simulink model "mini_car_ble"  (R2024a)
settings: Solver=FixedStepAuto  StartTime=0.0  StopTime=inf  FixedStep=0.02  RelTol=1e-3
undefined symbols (not defined in the file): u2, u3, u4, u5
libraries: simulink x57
settings Model: Creator=ext_matsmi1  LastModifiedBy=Matheus Smidi
settings OptimizationCC: DefaultParameterBehavior=Inlined  EnhancedBackFolding=on  PassReuseOutputArgsAs=Individual arguments  ZeroExternalMemoryAtStartup=off  ZeroInternalMemoryAtStartup=off  OptimizeBlockOrder=speed  DifferentSizesBufferReuse=on  OptimizationCustomize=off  EfficientTunableParamExpr=on
settings DebuggingCC: ParameterTunabilityLossMsg=error
settings HardwareCC: ProdHWDeviceType=AMD->x86-64 (Windows64)
settings SFSimCC: MATLABDynamicMemAlloc=off
settings RTWCC: Description=Embedded Coder  SystemTargetFile=ert.tlc  TemplateMakefile=ert_default_tmf  GPUComputeCapability=3.5
settings CodeAppCC: ForceParamTrailComments=on  IgnoreCustomStorageClasses=off  OperatorAnnotations=on  SimulinkDataObjDesc=on  SFDataObjDesc=on  InsertBlockDesc=on
settings ERTTargetCC: TargetLangStandard=C99 (ISO)  GenerateSampleERTMain=on  InlinedParameterPlacement=NonHierarchical  ERTCustomFileTemplate=example_file_process.tlc

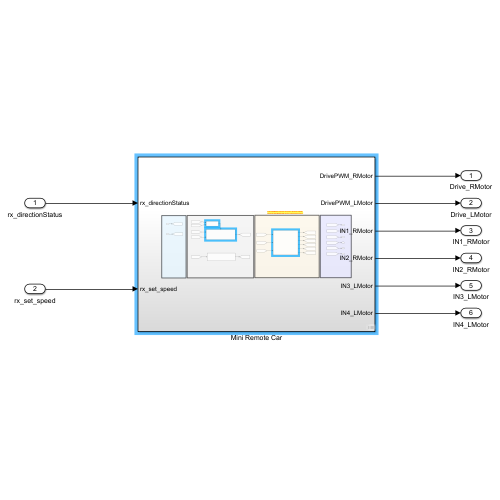
[thumbnail: Simulink's stored preview of the top-level diagram]
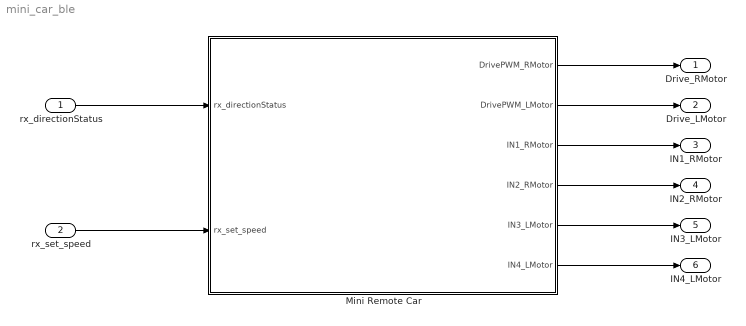
== system mini_car_ble ==
  rx_directionStatus : Inport  OutDataTypeStr=uint16
  rx_set_speed : Inport  Port=2  OutDataTypeStr=uint16
  Mini Remote Car : Subsystem
  Drive_RMotor : Outport
  Drive_LMotor : Outport  Port=2
  IN1_RMotor : Outport  Port=3
  IN2_RMotor : Outport  Port=4
  IN3_LMotor : Outport  Port=5
  IN4_LMotor : Outport  Port=6
  wires:
  Mini Remote Car/3(IN1_RMotor) -> IN1_RMotor/1
  Mini Remote Car/1(DrivePWM_RMotor) -> Drive_RMotor/1
  Mini Remote Car/6(IN4_LMotor) -> IN4_LMotor/1
  Mini Remote Car/4(IN2_RMotor) -> IN2_RMotor/1
  Mini Remote Car/5(IN3_LMotor) -> IN3_LMotor/1
  Mini Remote Car/2(DrivePWM_LMotor) -> Drive_LMotor/1
  rx_set_speed/1 -> Mini Remote Car/2(rx_set_speed)
  rx_directionStatus/1 -> Mini Remote Car/1(rx_directionStatus)

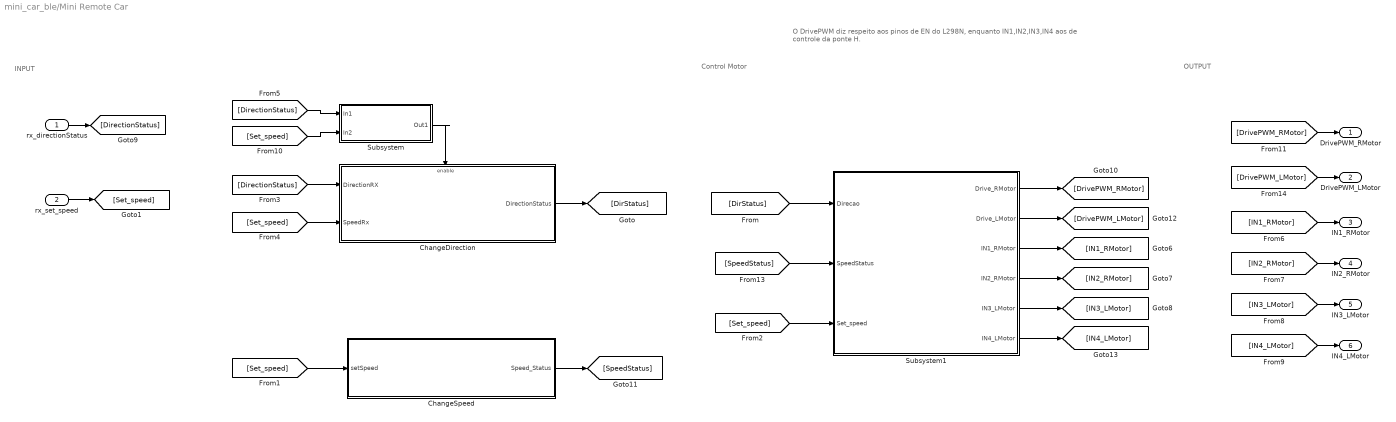
== system mini_car_ble/Mini Remote Car ==
  note: O DrivePWM diz respeito aos pinos de EN do L298N, enquanto IN1,IN2,IN3,IN4 aos de controle da ponte H.
  note: INPUT
  note: OUTPUT
  note: Control Motor
  rx_directionStatus : Inport
  rx_set_speed : Inport  Port=2
  ChangeDirection : Subsystem
  ChangeSpeed : Subsystem
  Subsystem : Subsystem
  Subsystem1 : Subsystem
  DrivePWM_RMotor : Outport
  DrivePWM_LMotor : Outport  Port=2
  IN1_RMotor : Outport  Port=3
  IN2_RMotor : Outport  Port=4
  IN3_LMotor : Outport  Port=5
  IN4_LMotor : Outport  Port=6
  wires:
  rx_directionStatus/1 -> [DirectionStatus]
  [DirStatus] -> Subsystem1/1(Direcao)
  Subsystem1/1(Drive_RMotor) -> [DrivePWM_RMotor]
  [DrivePWM_RMotor] -> DrivePWM_RMotor/1
  ChangeSpeed/1(Speed_Status) -> [SpeedStatus]
  [SpeedStatus] -> Subsystem1/2(SpeedStatus)
  Subsystem1/2(Drive_LMotor) -> [DrivePWM_LMotor]
  [DrivePWM_LMotor] -> DrivePWM_LMotor/1
  Subsystem1/3(IN1_RMotor) -> [IN1_RMotor]
  Subsystem1/4(IN2_RMotor) -> [IN2_RMotor]
  Subsystem1/5(IN3_LMotor) -> [IN3_LMotor]
  Subsystem1/6(IN4_LMotor) -> [IN4_LMotor]
  [IN1_RMotor] -> IN1_RMotor/1
  [IN2_RMotor] -> IN2_RMotor/1
  [IN3_LMotor] -> IN3_LMotor/1
  [IN4_LMotor] -> IN4_LMotor/1
  rx_set_speed/1 -> [Set_speed]
  [Set_speed] -> ChangeSpeed/1(setSpeed)
  [Set_speed] -> Subsystem1/3(Set_speed)
  [DirectionStatus] -> ChangeDirection/1(DirectionRX)
  [Set_speed] -> ChangeDirection/2(SpeedRx)
  ChangeDirection/1(DirectionStatus) -> [DirStatus]
  Subsystem/1(Out1) -> ChangeDirection/Enable
  [DirectionStatus] -> Subsystem/1(In1)
  [Set_speed] -> Subsystem/2(In2)

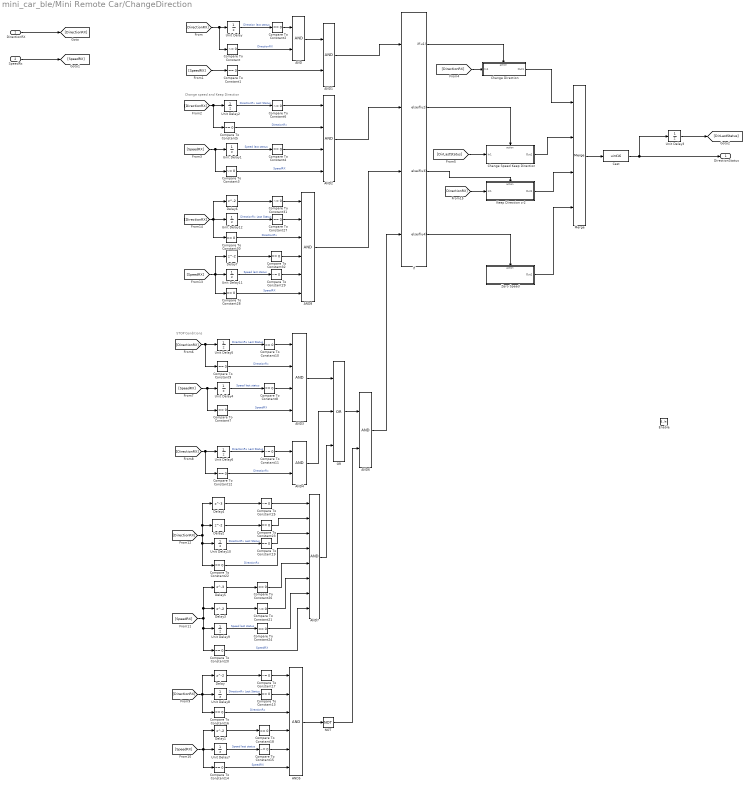
== system mini_car_ble/Mini Remote Car/ChangeDirection ==
  note: Change speed and Keep Direction
  note: STOP Conditions
  DirectionRX : Inport
  SpeedRx : Inport  Port=2
  Enable : EnablePort
  AND{,1,4,6} (4 alike) : Logic  AllPortsSameDT=off  OutDataTypeStr=boolean
  AND2 : Logic  Inputs=4  AllPortsSameDT=off  OutDataTypeStr=boolean
  AND3 : Logic  Inputs=4  AllPortsSameDT=off  OutDataTypeStr=boolean
  AND5 : Logic  Inputs=6  AllPortsSameDT=off  OutDataTypeStr=boolean
  AND7 : Logic  Inputs=8  AllPortsSameDT=off  OutDataTypeStr=boolean
  AND8 : Logic  Inputs=6  AllPortsSameDT=off  OutDataTypeStr=boolean
  Cast : DataTypeConversion  OutDataTypeStr=uint16  SaturateOnIntegerOverflow=off  RndMeth=Floor
  Change Direction : Subsystem  TreatAsAtomicUnit=on
  Change Speed Keep Direction : Subsystem  TreatAsAtomicUnit=on
  Compare To Constant{,3,6,11,15,17,21,25,29,31} (10 alike) : simulink/Logic and Bit Operations/Compare To Constant  relop=~=  const=0  OutDataTypeStr=boolean
  Compare To Constant{1..2,4..5,7..10,12..14,16,18..20,22..24,26..28,30,32} (23 alike) : simulink/Logic and Bit Operations/Compare To Constant  relop===  const=0  OutDataTypeStr=boolean
  Delay{,1..3,6..7} (6 alike) : Delay
  Delay4 : Delay  DelayLength=3
  Delay5 : Delay  DelayLength=3
  If : If  NumInputs=4  IfExpression=u1  ElseIfExpressions=u2,u3,u4  ShowElse=off
  Keep Direction z-2 : Subsystem  TreatAsAtomicUnit=on
  Merge : Merge  Inputs=4
  NOT : Logic  Operator=NOT  AllPortsSameDT=off  OutDataTypeStr=boolean
  OR : Logic  Operator=OR  Inputs=3  AllPortsSameDT=off  OutDataTypeStr=boolean
  Unit Delay{,1..12} (13 alike) : UnitDelay  SampleTime=-1  HasFrameUpgradeWarning=on
  Zero Speed : Subsystem  TreatAsAtomicUnit=on
  DirectionStatus : Outport
  wires:
  Compare To Constant/1 -> AND/2  "DirectionRX"
  AND/1 -> AND1/1
  Compare To Constant1/1 -> AND1/2
  AND1/1 -> If/1
  DirectionRX/1 -> [DirectionRX]
  SpeedRx/1 -> [SpeedRX]
  [DirectionRX] -> Unit Delay/1, Compare To Constant/1
  [SpeedRX] -> Compare To Constant1/1
  If/1 -> Change Direction/Action
  Compare To Constant3/1 -> AND2/4  "SpeedRX"
  [SpeedRX] -> Unit Delay1/1, Compare To Constant3/1
  [DirectionRX] -> Unit Delay2/1, Compare To Constant5/1
  Compare To Constant5/1 -> AND2/2  "DirectionRx"
  Unit Delay3/1 -> [DirLastStatus]
  [DirectionRX] -> Change Direction/1(In1)
  If/2 -> Change Speed Keep Direction/Action
  [DirLastStatus] -> Change Speed Keep Direction/1(In1)
  Change Direction/1(Out1) -> Merge/1
  Change Speed Keep Direction/1(Out1) -> Merge/2
  Compare To Constant9/1 -> AND3/2  "DirectionRx"
  Compare To Constant7/1 -> AND3/4  "SpeedRX"
  [DirectionRX] -> Unit Delay5/1, Compare To Constant9/1
  [SpeedRX] -> Unit Delay4/1, Compare To Constant7/1
  Unit Delay/1 -> Compare To Constant2/1  "Direction last status"
  Compare To Constant2/1 -> AND/1
  Unit Delay2/1 -> Compare To Constant6/1  "DirectionRx Last Status"
  Compare To Constant6/1 -> AND2/1
  Unit Delay1/1 -> Compare To Constant4/1  "Speed last status"
  Compare To Constant4/1 -> AND2/3
  Unit Delay5/1 -> Compare To Constant10/1  "DirectionRx Last Status"
  Compare To Constant10/1 -> AND3/1
  Unit Delay4/1 -> Compare To Constant8/1  "Speed last status"
  Compare To Constant8/1 -> AND3/3
  Unit Delay6/1 -> Compare To Constant11/1  "DirectionRx Last Status"
  [DirectionRX] -> Unit Delay6/1, Compare To Constant12/1
  AND3/1 -> OR/1
  Compare To Constant11/1 -> AND4/1
  Compare To Constant12/1 -> AND4/2  "DirectionRx"
  AND4/1 -> OR/2
  Merge/1 -> Cast/1
  Cast/1 -> Unit Delay3/1, DirectionStatus/1
  Unit Delay8/1 -> Compare To Constant13/1  "DirectionRx Last Status"
  [SpeedRX] -> Delay1/1, Unit Delay7/1, Compare To Constant14/1
  [DirectionRX] -> Unit Delay8/1, Compare To Constant16/1, Delay/1
  Delay/1 -> Compare To Constant17/1
  Unit Delay7/1 -> Compare To Constant15/1  "Speed last status"
  Delay1/1 -> Compare To Constant18/1
  Compare To Constant17/1 -> AND5/1
  Compare To Constant13/1 -> AND5/2
  Compare To Constant16/1 -> AND5/3  "DirectionRx"
  Compare To Constant18/1 -> AND5/4
  Compare To Constant15/1 -> AND5/5
  Compare To Constant14/1 -> AND5/6  "SpeedRX"
  AND5/1 -> NOT/1
  OR/1 -> AND6/1
  [DirectionRX] -> Delay4/1, Delay2/1, Unit Delay10/1, Compare To Constant22/1
  [SpeedRX] -> Delay5/1, Delay3/1, Unit Delay9/1, Compare To Constant20/1
  Compare To Constant20/1 -> AND7/8  "SpeedRX"
  Unit Delay10/1 -> Compare To Constant19/1  "DirectionRx Last Status"
  Delay2/1 -> Compare To Constant23/1
  Delay4/1 -> Compare To Constant25/1
  Unit Delay9/1 -> Compare To Constant24/1  "Speed last status"
  Delay3/1 -> Compare To Constant21/1
  Delay5/1 -> Compare To Constant26/1
  Compare To Constant25/1 -> AND7/1
  Compare To Constant23/1 -> AND7/2
  Compare To Constant19/1 -> AND7/3
  Compare To Constant22/1 -> AND7/4  "DirectionRx"
  Compare To Constant26/1 -> AND7/5
  Compare To Constant21/1 -> AND7/6
  Compare To Constant24/1 -> AND7/7
  AND7/1 -> OR/3
  NOT/1 -> AND6/2
  Unit Delay11/1 -> Compare To Constant29/1  "Speed last status"
  [SpeedRX] -> Delay7/1, Unit Delay11/1, Compare To Constant28/1
  Compare To Constant29/1 -> AND8/5
  Compare To Constant28/1 -> AND8/6  "SpeedRX"
  Compare To Constant31/1 -> AND8/1
  Compare To Constant30/1 -> AND8/3  "DirectionRx"
  Unit Delay12/1 -> Compare To Constant27/1  "DirectionRx Last Status"
  Compare To Constant27/1 -> AND8/2
  Compare To Constant32/1 -> AND8/4
  [DirectionRX] -> Unit Delay12/1, Compare To Constant30/1, Delay6/1
  Delay7/1 -> Compare To Constant32/1
  Delay6/1 -> Compare To Constant31/1
  AND2/1 -> If/2
  Zero Speed/1(Out1) -> Merge/4
  If/4 -> Zero Speed/Action
  AND8/1 -> If/3
  AND6/1 -> If/4
  If/3 -> Keep Direction z-2/Action
  Keep Direction z-2/1(Out1) -> Merge/3
  [DirectionRX] -> Keep Direction z-2/1(In1)

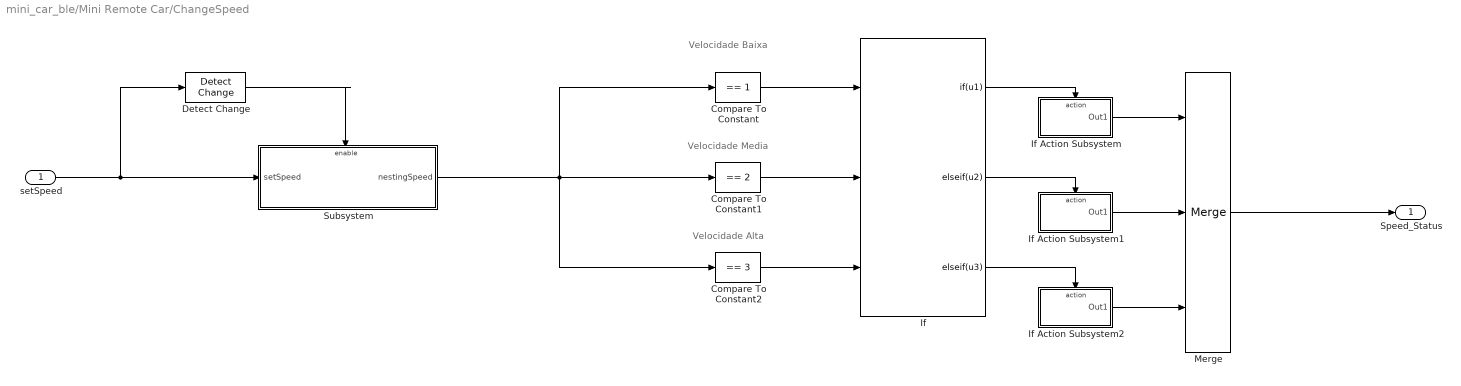
== system mini_car_ble/Mini Remote Car/ChangeSpeed ==
  note: Velocidade Alta
  note: Velocidade Media
  note: Velocidade Baixa
  setSpeed : Inport
  Compare To Constant : simulink/Logic and Bit Operations/Compare To Constant  relop===  const=1  OutDataTypeStr=boolean
  Compare To Constant1 : simulink/Logic and Bit Operations/Compare To Constant  relop===  const=2  OutDataTypeStr=boolean
  Compare To Constant2 : simulink/Logic and Bit Operations/Compare To Constant  relop===  const=3  OutDataTypeStr=boolean
  Detect Change : simulink/Logic and Bit Operations/Detect Change  vinit=0  OutDataTypeStr=boolean
  If : If  NumInputs=3  IfExpression=u1  ElseIfExpressions=u2,u3  ShowElse=off
  If Action Subsystem : Subsystem  TreatAsAtomicUnit=on
  If Action Subsystem1 : Subsystem  TreatAsAtomicUnit=on
  If Action Subsystem2 : Subsystem  TreatAsAtomicUnit=on
  Merge : Merge  Inputs=3
  Subsystem : Subsystem
  Speed_Status : Outport
  wires:
  If/1 -> If Action Subsystem/Action
  If Action Subsystem1/1(Out1) -> Merge/2
  If Action Subsystem/1(Out1) -> Merge/1
  If Action Subsystem2/1(Out1) -> Merge/3
  If/3 -> If Action Subsystem2/Action
  Compare To Constant/1 -> If/1
  If/2 -> If Action Subsystem1/Action
  Compare To Constant2/1 -> If/3
  Compare To Constant1/1 -> If/2
  Merge/1 -> Speed_Status/1
  setSpeed/1 -> Detect Change/1, Subsystem/1(setSpeed)
  Subsystem/1(nestingSpeed) -> Compare To Constant2/1, Compare To Constant/1, Compare To Constant1/1
  Detect Change/1 -> Subsystem/Enable

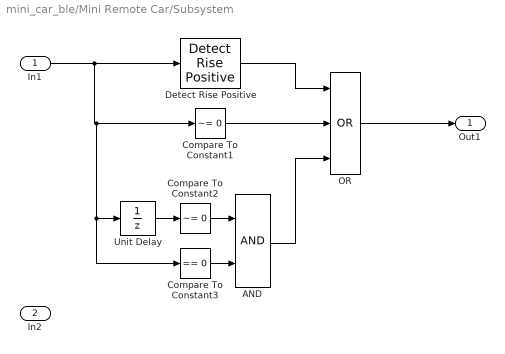
== system mini_car_ble/Mini Remote Car/Subsystem ==
  In1 : Inport
  In2 : Inport  Port=2
  AND : Logic  AllPortsSameDT=off  OutDataTypeStr=boolean
  Compare To Constant1 : simulink/Logic and Bit Operations/Compare To Constant  relop=~=  const=0  OutDataTypeStr=boolean
  Compare To Constant2 : simulink/Logic and Bit Operations/Compare To Constant  relop=~=  const=0  OutDataTypeStr=boolean
  Compare To Constant3 : simulink/Logic and Bit Operations/Compare To Constant  relop===  const=0  OutDataTypeStr=boolean
  Detect Rise Positive : simulink/Logic and Bit Operations/Detect Rise Positive  vinit=0  OutDataTypeStr=boolean
  OR : Logic  Operator=OR  Inputs=3  AllPortsSameDT=off  OutDataTypeStr=boolean
  Unit Delay : UnitDelay  SampleTime=-1  HasFrameUpgradeWarning=on
  Out1 : Outport
  wires:
  In1/1 -> Detect Rise Positive/1, Unit Delay/1, Compare To Constant3/1, Compare To Constant1/1
  Detect Rise Positive/1 -> OR/1
  Compare To Constant1/1 -> OR/2
  OR/1 -> Out1/1
  Unit Delay/1 -> Compare To Constant2/1
  Compare To Constant3/1 -> AND/2
  Compare To Constant2/1 -> AND/1
  AND/1 -> OR/3

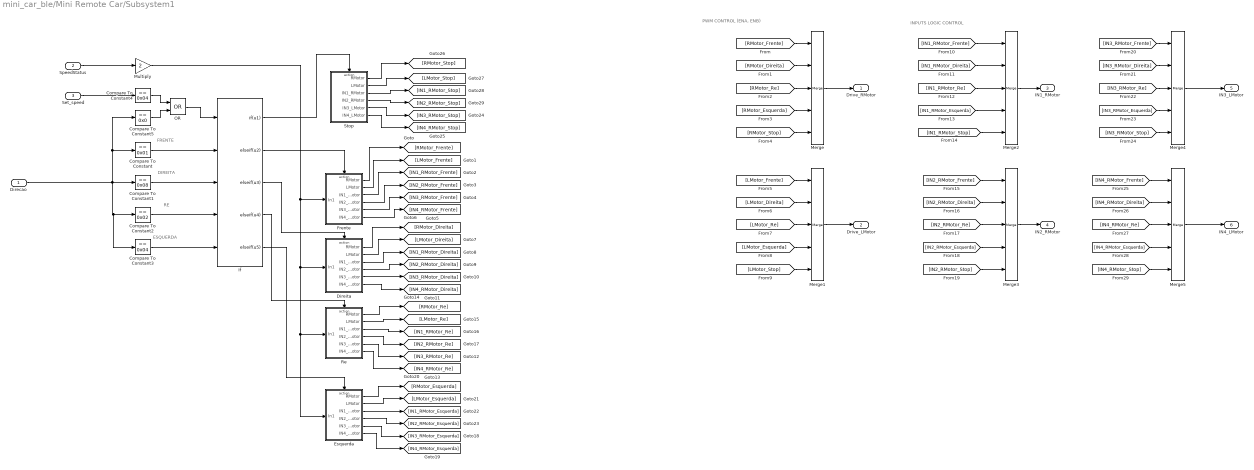
== system mini_car_ble/Mini Remote Car/Subsystem1 ==
  note: INPUTS LOGIC CONTROL
  note: PWM CONTROL (ENA, ENB)
  note: DIREITA
  note: ESQUERDA
  note: FRENTE
  note: RE
  Direcao : Inport
  SpeedStatus : Inport  Port=2
  Set_speed : Inport  Port=3
  Compare To Constant : simulink/Logic and Bit Operations/Compare To Constant  relop===  const=0x01  OutDataTypeStr=boolean
  Compare To Constant1 : simulink/Logic and Bit Operations/Compare To Constant  relop===  const=0x08  OutDataTypeStr=boolean
  Compare To Constant2 : simulink/Logic and Bit Operations/Compare To Constant  relop===  const=0x02  OutDataTypeStr=boolean
  Compare To Constant3 : simulink/Logic and Bit Operations/Compare To Constant  relop===  const=0x04  OutDataTypeStr=boolean
  Compare To Constant4 : simulink/Logic and Bit Operations/Compare To Constant  relop===  const=0x04  OutDataTypeStr=boolean
  Compare To Constant5 : simulink/Logic and Bit Operations/Compare To Constant  relop===  const=0x0  OutDataTypeStr=boolean
  Direita : Subsystem  TreatAsAtomicUnit=on
  Esquerda : Subsystem  TreatAsAtomicUnit=on
  Frente : Subsystem  TreatAsAtomicUnit=on
  If : If  NumInputs=5  IfExpression=u1  ElseIfExpressions=u2,u3,u4,u5  ShowElse=off
  Merge{,1..5} (6 alike) : Merge  Inputs=5
  Multiply : Gain  Gain=2
  OR : Logic  Operator=OR  AllPortsSameDT=off  OutDataTypeStr=boolean
  Re : Subsystem  TreatAsAtomicUnit=on
  Stop : Subsystem  TreatAsAtomicUnit=on
  Drive_RMotor : Outport
  Drive_LMotor : Outport  Port=2
  IN1_RMotor : Outport  Port=3
  IN2_RMotor : Outport  Port=4
  IN3_LMotor : Outport  Port=5
  IN4_LMotor : Outport  Port=6
  wires:
  Merge/1 -> Drive_RMotor/1
  Merge1/1 -> Drive_LMotor/1
  Merge2/1 -> IN1_RMotor/1
  Merge3/1 -> IN2_RMotor/1
  Merge4/1 -> IN3_LMotor/1
  Merge5/1 -> IN4_LMotor/1
  [RMotor_Frente] -> Merge/1
  [RMotor_Direita] -> Merge/2
  [RMotor_Re] -> Merge/3
  [RMotor_Esquerda] -> Merge/4
  [RMotor_Stop] -> Merge/5
  [LMotor_Frente] -> Merge1/1
  [LMotor_Direita] -> Merge1/2
  [LMotor_Re] -> Merge1/3
  [LMotor_Esquerda] -> Merge1/4
  [LMotor_Stop] -> Merge1/5
  [IN1_RMotor_Frente] -> Merge2/1
  [IN1_RMotor_Direita] -> Merge2/2
  [IN1_RMotor_Stop] -> Merge2/5
  [IN1_RMotor_Esquerda] -> Merge2/4
  [IN1_RMotor_Re] -> Merge2/3
  [IN2_RMotor_Frente] -> Merge3/1
  [IN2_RMotor_Direita] -> Merge3/2
  [IN2_RMotor_Re] -> Merge3/3
  [IN2_RMotor_Esquerda] -> Merge3/4
  [IN2_RMotor_Stop] -> Merge3/5
  [IN3_RMotor_Frente] -> Merge4/1
  [IN3_RMotor_Direita] -> Merge4/2
  [IN3_RMotor_Re] -> Merge4/3
  [IN3_RMotor_Esquerda] -> Merge4/4
  [IN3_RMotor_Stop] -> Merge4/5
  [IN4_RMotor_Frente] -> Merge5/1
  [IN4_RMotor_Direita] -> Merge5/2
  [IN4_RMotor_Re] -> Merge5/3
  [IN4_RMotor_Esquerda] -> Merge5/4
  [IN4_RMotor_Stop] -> Merge5/5
  Stop/3(IN1_RMotor) -> [IN1_RMotor_Stop]
  Stop/1(RMotor) -> [RMotor_Stop]
  Stop/2(LMotor) -> [LMotor_Stop]
  Esquerda/6(IN4_LMotor) -> [IN4_RMotor_Esquerda]
  Stop/6(IN4_LMotor) -> [IN4_RMotor_Stop]
  Stop/5(IN3_LMotor) -> [IN3_RMotor_Stop]
  Esquerda/2(LMotor) -> [LMotor_Esquerda]
  Direita/5(IN3_LMotor) -> [IN3_RMotor_Direita]
  Re/1(RMotor) -> [RMotor_Re]
  Direita/4(IN2_RMotor) -> [IN2_RMotor_Direita]
  Direita/1(RMotor) -> [RMotor_Direita]
  Esquerda/4(IN2_RMotor) -> [IN2_RMotor_Esquerda]
  Re/2(LMotor) -> [LMotor_Re]
  Esquerda/1(RMotor) -> [RMotor_Esquerda]
  Direita/6(IN4_LMotor) -> [IN4_RMotor_Direita]
  Frente/4(IN2_RMotor) -> [IN2_RMotor_Frente]
  Frente/1(RMotor) -> [RMotor_Frente]
  Frente/3(IN1_RMotor) -> [IN1_RMotor_Frente]
  SpeedStatus/1 -> Multiply/1
  Frente/6(IN4_LMotor) -> [IN4_RMotor_Frente]
  Frente/5(IN3_LMotor) -> [IN3_RMotor_Frente]
  Esquerda/5(IN3_LMotor) -> [IN3_RMotor_Esquerda]
  Multiply/1 -> Esquerda/1(In1), Re/1(In1), Direita/1(In1), Frente/1(In1)
  Re/6(IN4_LMotor) -> [IN4_RMotor_Re]
  Direita/3(IN1_RMotor) -> [IN1_RMotor_Direita]
  Re/3(IN1_RMotor) -> [IN1_RMotor_Re]
  Direita/2(LMotor) -> [LMotor_Direita]
  Esquerda/3(IN1_RMotor) -> [IN1_RMotor_Esquerda]
  Stop/4(IN2_RMotor) -> [IN2_RMotor_Stop]
  Re/4(IN2_RMotor) -> [IN2_RMotor_Re]
  Re/5(IN3_LMotor) -> [IN3_RMotor_Re]
  Direcao/1 -> Compare To Constant1/1, Compare To Constant3/1, Compare To Constant2/1, Compare To Constant5/1, Compare To Constant/1
  Frente/2(LMotor) -> [LMotor_Frente]
  Compare To Constant3/1 -> If/5
  Compare To Constant2/1 -> If/4
  Compare To Constant1/1 -> If/3
  Compare To Constant/1 -> If/2
  Set_speed/1 -> Compare To Constant4/1
  If/1 -> Stop/Action
  If/2 -> Frente/Action
  If/3 -> Direita/Action
  If/4 -> Re/Action
  If/5 -> Esquerda/Action
  Compare To Constant4/1 -> OR/1
  Compare To Constant5/1 -> OR/2
  OR/1 -> If/1

== system mini_car_ble/Mini Remote Car/ChangeDirection/Change Direction ==
  In1 : Inport
  Action Port : ActionPort  ActionPortLabel=if(u1)
  Out1 : Outport
  wires:
  In1/1 -> Out1/1

== system mini_car_ble/Mini Remote Car/ChangeDirection/Change Speed Keep Direction ==
  In1 : Inport
  Action Port : ActionPort  ActionPortLabel=elseif(u2)
  Out1 : Outport
  wires:
  In1/1 -> Out1/1

== system mini_car_ble/Mini Remote Car/ChangeDirection/Keep Direction z-2 ==
  In1 : Inport
  Action Port : ActionPort  ActionPortLabel=elseif(u3)
  Delay : Delay
  Out1 : Outport
  wires:
  Delay/1 -> Out1/1
  In1/1 -> Delay/1

== system mini_car_ble/Mini Remote Car/ChangeDirection/Zero Speed ==
  Action Port : ActionPort  ActionPortLabel=elseif(u4)
  Constant : Constant  Value=0  OutDataTypeStr=uint16
  Out1 : Outport
  wires:
  Constant/1 -> Out1/1

== system mini_car_ble/Mini Remote Car/ChangeSpeed/If Action Subsystem ==
  Action Port : ActionPort  ActionPortLabel=if(u1)
  Constant : Constant  Value=420
  Out1 : Outport
  wires:
  Constant/1 -> Out1/1

== system mini_car_ble/Mini Remote Car/ChangeSpeed/If Action Subsystem1 ==
  Action Port : ActionPort  ActionPortLabel=elseif(u2)
  Constant : Constant  Value=450
  Out1 : Outport
  wires:
  Constant/1 -> Out1/1

== system mini_car_ble/Mini Remote Car/ChangeSpeed/If Action Subsystem2 ==
  Action Port : ActionPort  ActionPortLabel=elseif(u3)
  Constant : Constant  Value=500
  Out1 : Outport
  wires:
  Constant/1 -> Out1/1

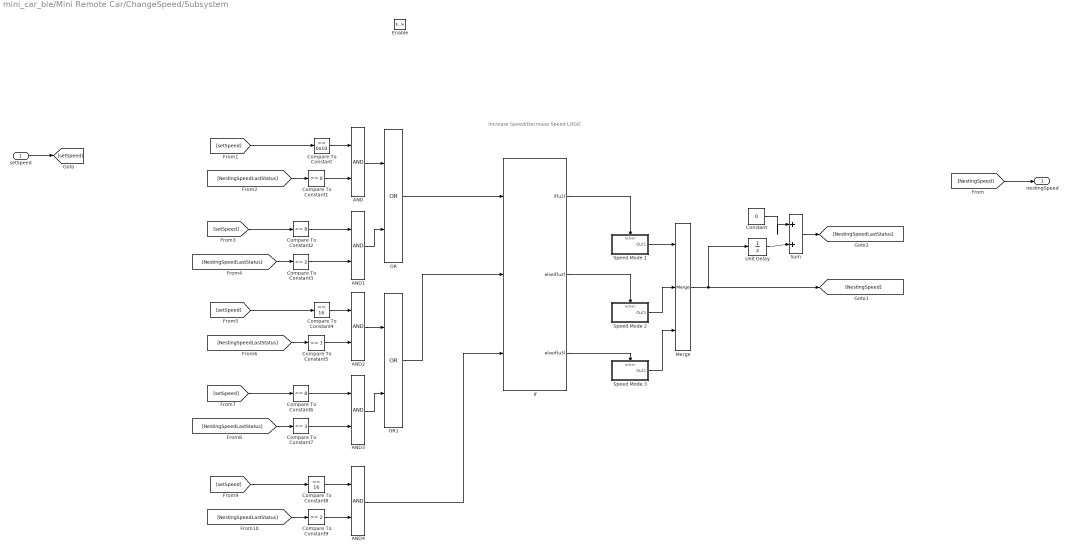
== system mini_car_ble/Mini Remote Car/ChangeSpeed/Subsystem ==
  note: Increase Speed/Decrease Speed LOGIC
  setSpeed : Inport
  Enable : EnablePort
  AND{,1..4} (5 alike) : Logic  AllPortsSameDT=off  OutDataTypeStr=boolean
  Compare To Constant : simulink/Logic and Bit Operations/Compare To Constant  relop===  const=0x10  OutDataTypeStr=boolean
  Compare To Constant1 : simulink/Logic and Bit Operations/Compare To Constant  relop===  const=0  OutDataTypeStr=boolean
  Compare To Constant2 : simulink/Logic and Bit Operations/Compare To Constant  relop===  const=8  OutDataTypeStr=boolean
  Compare To Constant3 : simulink/Logic and Bit Operations/Compare To Constant  relop===  const=2  OutDataTypeStr=boolean
  Compare To Constant4 : simulink/Logic and Bit Operations/Compare To Constant  relop===  const=16  OutDataTypeStr=boolean
  Compare To Constant5 : simulink/Logic and Bit Operations/Compare To Constant  relop===  const=1  OutDataTypeStr=boolean
  Compare To Constant6 : simulink/Logic and Bit Operations/Compare To Constant  relop===  const=8  OutDataTypeStr=boolean
  Compare To Constant7 : simulink/Logic and Bit Operations/Compare To Constant  relop===  const=3  OutDataTypeStr=boolean
  Compare To Constant8 : simulink/Logic and Bit Operations/Compare To Constant  relop===  const=16  OutDataTypeStr=boolean
  Compare To Constant9 : simulink/Logic and Bit Operations/Compare To Constant  relop===  const=2  OutDataTypeStr=boolean
  Constant : Constant  Value=0  OutDataTypeStr=uint16
  If : If  NumInputs=3  IfExpression=u1  ElseIfExpressions=u2,u3  ShowElse=off
  Merge : Merge  Inputs=3
  OR : Logic  Operator=OR  AllPortsSameDT=off  OutDataTypeStr=boolean
  OR1 : Logic  Operator=OR  AllPortsSameDT=off  OutDataTypeStr=boolean
  Speed Mode 1 : Subsystem  TreatAsAtomicUnit=on
  Speed Mode 2 : Subsystem  TreatAsAtomicUnit=on
  Speed Mode 3 : Subsystem  TreatAsAtomicUnit=on
  Sum : Sum  Inputs=|++
  Unit Delay : UnitDelay  SampleTime=-1  HasFrameUpgradeWarning=on
  nestingSpeed : Outport
  wires:
  setSpeed/1 -> [setSpeed]
  [setSpeed] -> Compare To Constant/1
  If/1 -> Speed Mode 1/Action
  Merge/1 -> [NestingSpeed], Unit Delay/1
  Speed Mode 1/1(Out1) -> Merge/1
  Speed Mode 2/1(Out1) -> Merge/2
  Speed Mode 3/1(Out1) -> Merge/3
  If/2 -> Speed Mode 2/Action
  If/3 -> Speed Mode 3/Action
  [NestingSpeedLastStatus] -> Compare To Constant1/1
  Compare To Constant/1 -> AND/1
  Compare To Constant1/1 -> AND/2
  [setSpeed] -> Compare To Constant2/1
  Compare To Constant2/1 -> AND1/1
  [NestingSpeedLastStatus] -> Compare To Constant3/1
  Compare To Constant3/1 -> AND1/2
  AND/1 -> OR/1
  AND1/1 -> OR/2
  OR/1 -> If/1
  AND2/1 -> OR1/1
  [NestingSpeedLastStatus] -> Compare To Constant5/1
  [setSpeed] -> Compare To Constant6/1
  Compare To Constant7/1 -> AND3/2
  AND3/1 -> OR1/2
  Compare To Constant6/1 -> AND3/1
  [NestingSpeedLastStatus] -> Compare To Constant7/1
  [setSpeed] -> Compare To Constant4/1
  Compare To Constant5/1 -> AND2/2
  Compare To Constant4/1 -> AND2/1
  OR1/1 -> If/2
  AND4/1 -> If/3
  [NestingSpeedLastStatus] -> Compare To Constant9/1
  [setSpeed] -> Compare To Constant8/1
  Compare To Constant9/1 -> AND4/2
  Compare To Constant8/1 -> AND4/1
  [NestingSpeed] -> nestingSpeed/1
  Sum/1 -> [NestingSpeedLastStatus]
  Constant/1 -> Sum/1
  Unit Delay/1 -> Sum/2

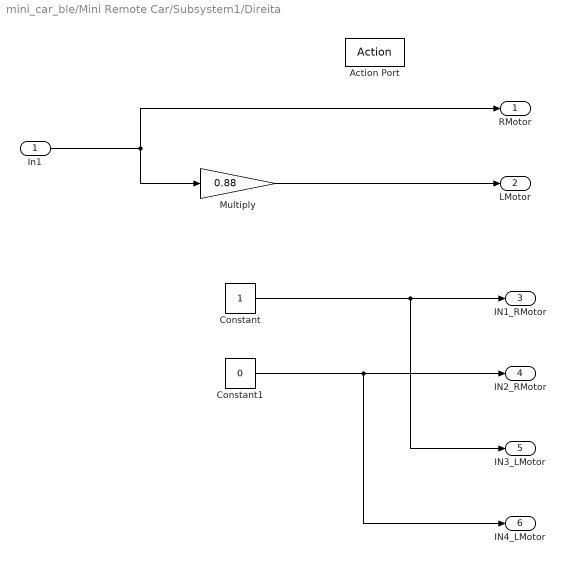
== system mini_car_ble/Mini Remote Car/Subsystem1/Direita ==
  In1 : Inport
  Action Port : ActionPort  ActionPortLabel=elseif(u3)
  Constant : Constant
  Constant1 : Constant  Value=0
  Multiply : Gain  Gain=0.88
  RMotor : Outport
  LMotor : Outport  Port=2
  IN1_RMotor : Outport  Port=3
  IN2_RMotor : Outport  Port=4
  IN3_LMotor : Outport  Port=5
  IN4_LMotor : Outport  Port=6
  wires:
  Multiply/1 -> LMotor/1
  In1/1 -> Multiply/1, RMotor/1
  Constant/1 -> IN3_LMotor/1, IN1_RMotor/1
  Constant1/1 -> IN4_LMotor/1, IN2_RMotor/1

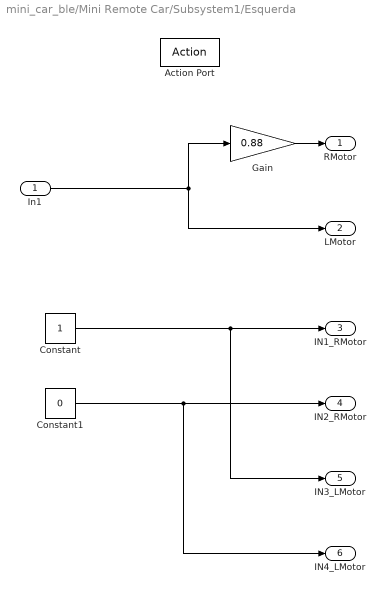
== system mini_car_ble/Mini Remote Car/Subsystem1/Esquerda ==
  In1 : Inport
  Action Port : ActionPort  ActionPortLabel=elseif(u5)
  Constant : Constant
  Constant1 : Constant  Value=0
  Gain : Gain  Gain=0.88
  RMotor : Outport
  LMotor : Outport  Port=2
  IN1_RMotor : Outport  Port=3
  IN2_RMotor : Outport  Port=4
  IN3_LMotor : Outport  Port=5
  IN4_LMotor : Outport  Port=6
  wires:
  In1/1 -> LMotor/1, Gain/1
  Gain/1 -> RMotor/1
  Constant/1 -> IN3_LMotor/1, IN1_RMotor/1
  Constant1/1 -> IN4_LMotor/1, IN2_RMotor/1

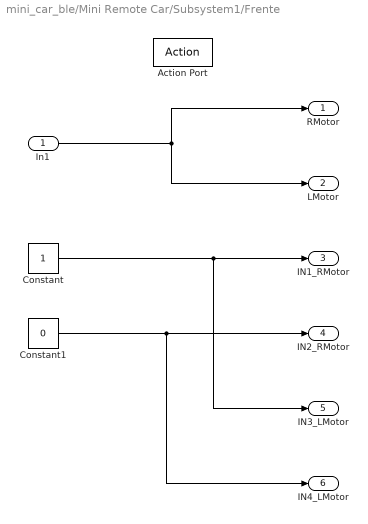
== system mini_car_ble/Mini Remote Car/Subsystem1/Frente ==
  In1 : Inport
  Action Port : ActionPort  ActionPortLabel=elseif(u2)
  Constant : Constant
  Constant1 : Constant  Value=0
  RMotor : Outport
  LMotor : Outport  Port=2
  IN1_RMotor : Outport  Port=3
  IN2_RMotor : Outport  Port=4
  IN3_LMotor : Outport  Port=5
  IN4_LMotor : Outport  Port=6
  wires:
  In1/1 -> RMotor/1, LMotor/1
  Constant/1 -> IN3_LMotor/1, IN1_RMotor/1
  Constant1/1 -> IN4_LMotor/1, IN2_RMotor/1

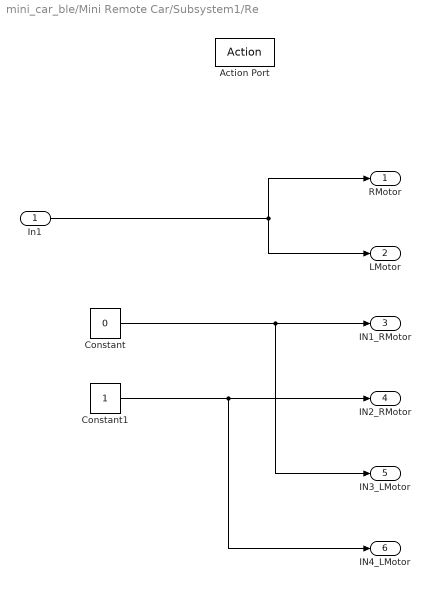
== system mini_car_ble/Mini Remote Car/Subsystem1/Re ==
  In1 : Inport
  Action Port : ActionPort  ActionPortLabel=elseif(u4)
  Constant : Constant  Value=0
  Constant1 : Constant
  RMotor : Outport
  LMotor : Outport  Port=2
  IN1_RMotor : Outport  Port=3
  IN2_RMotor : Outport  Port=4
  IN3_LMotor : Outport  Port=5
  IN4_LMotor : Outport  Port=6
  wires:
  In1/1 -> RMotor/1, LMotor/1
  Constant/1 -> IN3_LMotor/1, IN1_RMotor/1
  Constant1/1 -> IN4_LMotor/1, IN2_RMotor/1

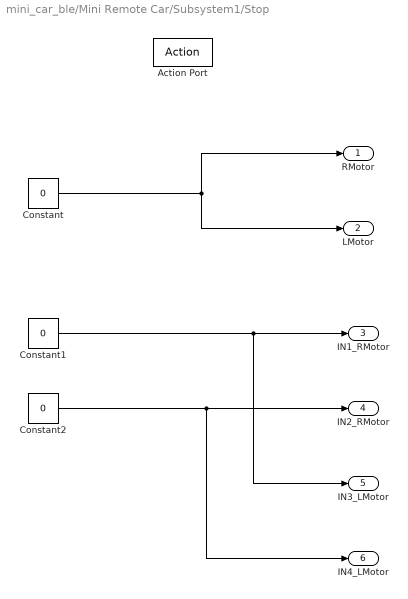
== system mini_car_ble/Mini Remote Car/Subsystem1/Stop ==
  Action Port : ActionPort  ActionPortLabel=if(u1)
  Constant : Constant  Value=0
  Constant1 : Constant  Value=0
  Constant2 : Constant  Value=0
  RMotor : Outport
  LMotor : Outport  Port=2
  IN1_RMotor : Outport  Port=3
  IN2_RMotor : Outport  Port=4
  IN3_LMotor : Outport  Port=5
  IN4_LMotor : Outport  Port=6
  wires:
  Constant/1 -> RMotor/1, LMotor/1
  Constant1/1 -> IN3_LMotor/1, IN1_RMotor/1
  Constant2/1 -> IN4_LMotor/1, IN2_RMotor/1

== system mini_car_ble/Mini Remote Car/ChangeSpeed/Subsystem/Speed Mode 1 ==
  Action Port : ActionPort  ActionPortLabel=if(u1)
  Constant : Constant  OutDataTypeStr=uint16
  Out1 : Outport
  wires:
  Constant/1 -> Out1/1

== system mini_car_ble/Mini Remote Car/ChangeSpeed/Subsystem/Speed Mode 2 ==
  Action Port : ActionPort  ActionPortLabel=elseif(u2)
  Constant : Constant  Value=2  OutDataTypeStr=uint16
  Out1 : Outport
  wires:
  Constant/1 -> Out1/1

== system mini_car_ble/Mini Remote Car/ChangeSpeed/Subsystem/Speed Mode 3 ==
  Action Port : ActionPort  ActionPortLabel=elseif(u3)
  Constant : Constant  Value=3  OutDataTypeStr=uint16
  Out1 : Outport
  wires:
  Constant/1 -> Out1/1
